simulink model "PolePlacement_Discrete"  (R2021a)
settings: Solver=VariableStepAuto  StartTime=0.0  StopTime=10.0  RelTol=1e-3
values from neighbouring files (symbols this model uses):
  k = place(A, B, new_pole)    [PolePlacement_Controller_script.m]
  k2 = place(sysest.A, sysest.B, new_pole2)    [PolePlacement_Controller_script.m]
  Kr = 1/Kdc(1)    [PolePlacement_Controller_script.m]
  Kr2 = 1/Kdc2    [PolePlacement_Controller_script.m]
  L = place(sysestc.A',sysestc.C', 10*new_pole)'    [PolePlacement_Controller_script.m]
  L22 = place(sysest.A',sysest.C', new_pole2/0.99)'    [PolePlacement_Controller_script.m]
  sysest = load("sysest09c_trick.mat").sysest    [Compensator_schemes.m]    (also in LQGR_Controller_script.m; PolePlacement_Controller_script.m)
undefined symbols (not defined in the file or in its folder): DiscIntNeverNeededParam, sigbuilder_block, sysestc
libraries: cstblocks x2, slpidlib x1
settings Model: Creator=jesuc  LastModifiedBy=andre

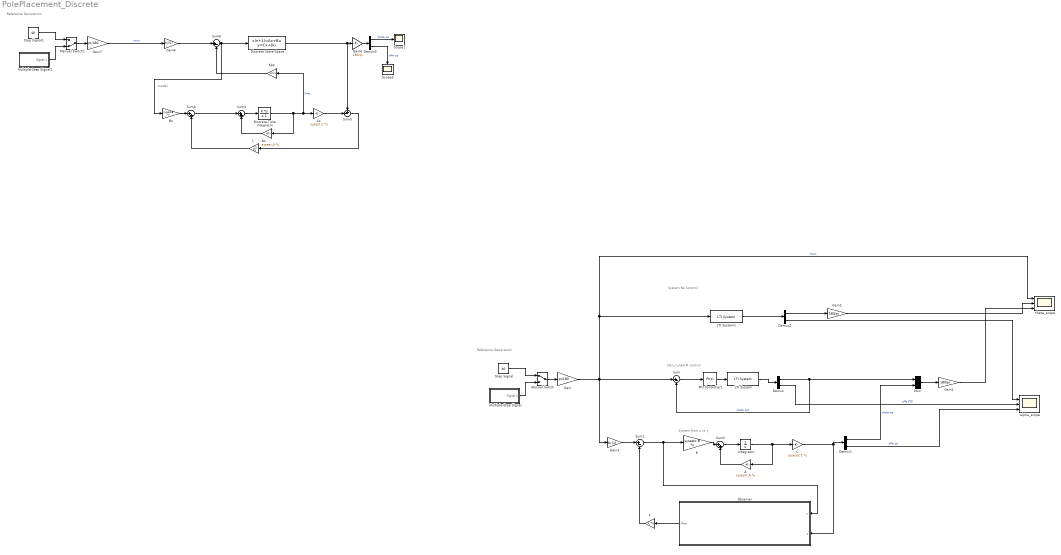
== system PolePlacement_Discrete ==
  note: Non_tuned PI control
  note: System No Control
  note: Reference Generation
  note: System from u to y
  note: model
  note: Reference Generation
  A : Gain  Gain=sysestc.A  Multiplication=Matrix(K*u)
  Ao : Gain  Gain=sysest.A  Multiplication=Matrix(K*u)
  B : Gain  Gain=sysestc.B  Multiplication=Matrix(K*u)
  Bo : Gain  Gain=sysest.B  Multiplication=Matrix(K*u)
  C : Gain  Gain=sysestc.C  Multiplication=Matrix(K*u)
  Co : Gain  Gain=sysest.C  Multiplication=Matrix(K*u)
  Demux{,1..3} (4 alike) : Demux  Outputs=2
  Discrete State-Space : DiscreteStateSpace  A=sysest.A  B=sysest.B  C=sysest.C  D=sysest.D  SampleTime=0.002
  Discrete-Time Integrator : DiscreteIntegrator  SampleTime=0.002  ICPrevOutput=DiscIntNeverNeededParam  ICPrevScaledInput=DiscIntNeverNeededParam
  Gain : Gain  Gain=pi/180
  Gain1 : Gain  Gain=180/pi
  Gain2 : Gain  Gain=180/pi
  Gain3 : Gain  Gain=Kr(1)
  Gain4 : Gain  Gain=Kr2(1)
  Gain6 : Gain  Gain=180/pi
  Gain7 : Gain  Gain=pi/180
  Integrator : Integrator
  K : Gain  Gain=k  Multiplication=Matrix(K*u)
  Kpp : Gain  Gain=k2  Multiplication=Matrix(K*u)
  L : Gain  Gain=L22  Multiplication=Matrix(K*u)
  LTI System : cstblocks/LTI System  sys=tf(sysestc)  IC=[]
  LTI System1 : cstblocks/LTI System  sys=tf(sysestc)  IC=[]
  Manual Switch : ManualSwitch
  Manual Switch1 : ManualSwitch  CurrentSetting=0
  Multiple-Step Signal : Subsystem  Tag=STV Subsys  LoadFcn=sigbuilder_block('load');  StartFcn=sigbuilder_block('start');  StopFcn=sigbuilder_block('stop');  ClipboardFcn=sigbuilder_block('clipboard');  mask(Sigbuilder block){tuvar=[0:10]}
      mask help: Simulink:masks:SigbuilderBlock_MD
      mask init:
      | if ~strcmp(get_param(bdroot(gcbh),'SimulationStatus'),'stopped') tuvar = sigbuilder_block('maskInit'); end
      settings: CopyFcn=sigbuilder_block('copy');  DeleteFcn=sigbuilder_block('delete');  ModelCloseFcn=sigbuilder_block('modelClose');  PreSaveFcn=sigbuilder_block('preSave');  PauseFcn=sigbuilder_block('pause');  ContinueFcn=sigbuilder_block('continue');  NameChangeFcn=sigbuilder_block('namechange');  OpenFcn=sigbuilder_block('open',[437.6 199.2 550.4 400 ]);  CloseFcn=sigbuilder_block('close');
      mask Display: plot(0, 0, 100, 100,[2, 2, 32, 32, 2], [68, 8, 8, 68, 68],[32, 2], [38, 38], [32, 19, 2],[53, 60, 44], [32, 17, 17, 2],[16, 16, 31, 31]);txt = getActiveGroup(gcbh);text(2, 100, txt,'verticalAlignment', 'top');
  Multiple-Step Signal1 : Subsystem  Tag=STV Subsys  LoadFcn=sigbuilder_block('load');  StartFcn=sigbuilder_block('start');  StopFcn=sigbuilder_block('stop');  ClipboardFcn=sigbuilder_block('clipboard');  mask(Sigbuilder block){tuvar=[0:10]}
      mask help: Simulink:masks:SigbuilderBlock_MD
      mask init:
      | if ~strcmp(get_param(bdroot(gcbh),'SimulationStatus'),'stopped') tuvar = sigbuilder_block('maskInit'); end
      settings: CopyFcn=sigbuilder_block('copy');  DeleteFcn=sigbuilder_block('delete');  ModelCloseFcn=sigbuilder_block('modelClose');  PreSaveFcn=sigbuilder_block('preSave');  PauseFcn=sigbuilder_block('pause');  ContinueFcn=sigbuilder_block('continue');  NameChangeFcn=sigbuilder_block('namechange');  OpenFcn=sigbuilder_block('open',[437.6 199.2 550.4 400 ]);  CloseFcn=sigbuilder_block('close');
      mask Display: plot(0, 0, 100, 100,[2, 2, 32, 32, 2], [68, 8, 8, 68, 68],[32, 2], [38, 38], [32, 19, 2],[53, 60, 44], [32, 17, 17, 2],[16, 16, 31, 31]);txt = getActiveGroup(gcbh);text(2, 100, txt,'verticalAlignment', 'top');
  Mux : Mux  Inputs=2
  Observer : Subsystem
  PID Controller1 : slpidlib/PID Controller  Controller=PI  Form=Parallel  TimeDomain=Continuous-time  UseExternalTs=off  SampleTime=-1  IntegratorMethod=Forward Euler  FilterMethod=Forward Euler  ControllerParametersSource=internal  P=1  I=1  D=0  UseFilter=on  N=100  TunerSelectOption=Transfer Function Based (PID Tuner App)  InitialConditionSource=internal  InitialConditionForIntegrator=0  InitialConditionForFilter=0  DifferentiatorICPrevScaledInput=0  ExternalReset=none  TrackingMode=off  Kt=1  LimitOutput=off  SatLimitsSource=internal  UpperSaturationLimit=inf  LowerSaturationLimit=-inf  LinearizeAsGain=on  AntiWindupMode=none  Kb=1  POutMin=[]  POutMax=[]  IOutMin=[]  IOutMax=[]  DOutMin=[]  DOutMax=[]  NOutMin=[]  NOutMax=[]  SumOutMin=[]  SumOutMax=[]  SaturationOutMin=[]  SaturationOutMax=[]  PParamMin=[]  PParamMax=[]  IParamMin=[]  IParamMax=[]  DParamMin=[]  DParamMax=[]  NParamMin=[]  NParamMax=[]  KbParamMin=[]  KbParamMax=[]  KtParamMin=[]  KtParamMax=[]  KbOutMin=[]  KbOutMax=[]  KtOutMin=[]  KtOutMax=[]  IntegratorOutMin=[]  IntegratorOutMax=[]  FilterOutMin=[]  FilterOutMax=[]  SumI1OutMin=[]  SumI1OutMax=[]  SumI2OutMin=[]  SumI2OutMax=[]  SumI3OutMin=[]  SumI3OutMax=[]  SumI4OutMin=[]  SumI4OutMax=[]  SumDOutMin=[]  SumDOutMax=[]  DifferentiatorOutMin=[]  DifferentiatorOutMax=[]  FilterDiffOutCoefMin=[]  FilterDiffOutCoefMax=[]  ReciprocalOutMin=[]  ReciprocalOutMax=[]  SumDenOutMin=[]  SumDenOutMax=[]  SumNumOutMin=[]  SumNumOutMax=[]  DivideOutMin=[]  DivideOutMax=[]  UdiffTsProdOutMin=[]  UdiffTsProdOutMax=[]  NTsProdOutMin=[]  NTsProdOutMax=[]  UintegralTsProdOutMin=[]  UintegralTsProdOutMax=[]  UngainTsProdOutMin=[]  UngainTsProdOutMax=[]  IntegratorContinuousStateAttributes=''  IntegratorStateMustResolveToSignalObject=off  IntegratorRTWStateStorageClass=Auto  FilterContinuousStateAttributes=''  FilterStateMustResolveToSignalObject=off  FilterRTWStateStorageClass=Auto  ParallelPVariant=InternalParameters  IdealPVariant=Disabled  IVariant=InternalParameters  DVariant=Disabled  IntegratorVariant=Continuous  SatVariant=Disabled  AWVariant=Passthrough  PCopyVariant=Disabled  TRVariant=Disabled  FdbkBlocksVariant=Forward  IdealPFdbkVariant=Disabled  SatFdbkVariant=Disabled  DerivativeFilterVariant=Disabled  NVariant=Disabled  NCopyVariant=Disabled_SignalSpec  FilterICVariant=Disabled  IntegratorICVariant=InternalICs  ExternalResetVariant=Disabled  TRSumVariant=Passthrough  SumFdbkVariant=Disabled  SumVariant=Sum_PI  TsampFilterVariant=InternalTs  TsampNgainVariant=Passthrough  TsampIntegralVariant=Passthrough  ExternalSaturationOutDataTypeStr=Inherit: Same as second input
  Scope1 : Scope
  Scope3 : Scope
  Step Signal : Constant  Value=40
  Step Signal1 : Constant  Value=40
  Sum : Sum  Inputs=|+-
  Sum1 : Sum  Inputs=|+-
  Sum2 : Sum  Inputs=|++
  Sum3 : Sum  Inputs=|++
  Sum4 : Sum  Inputs=|++
  Sum5 : Sum  Inputs=+-|
  Sum6 : Sum  Inputs=|+-
  alpha_scope : Scope  NumInputPorts=3
  theta_scope : Scope  NumInputPorts=3
  wires:
  Gain/1 -> theta_scope/1, LTI System1/1, Sum/1, Gain3/1  "input"
  Sum/1 -> PID Controller1/1
  PID Controller1/1 -> LTI System/1
  LTI System/1 -> Demux/1
  Demux/1 -> Sum/2, Mux/1  "theta pid"
  B/1 -> Sum2/1
  Sum2/1 -> Integrator/1
  Integrator/1 -> A/1, C/1
  A/1 -> Sum2/2
  K/1 -> Sum1/2
  C/1 -> Demux1/1, Observer/2(y)
  Demux1/1 -> Mux/2  "theta pp"
  Demux1/2 -> alpha_scope/3  "alfa pp"
  Gain3/1 -> Sum1/1
  Demux/2 -> alpha_scope/2  "alfa PID"
  Gain1/1 -> theta_scope/3
  Mux/1 -> Gain1/1
  Sum1/1 -> Observer/1(u), B/1
  Observer/1(Xhat) -> K/1
  LTI System1/1 -> Demux2/1
  Demux2/1 -> Gain2/1
  Gain2/1 -> theta_scope/2
  Demux2/2 -> alpha_scope/1
  Demux3/1 -> Scope1/1  "theta pp"
  Kpp/1 -> Sum6/2
  Sum4/1 -> Sum3/1
  Sum3/1 -> Discrete-Time Integrator/1
  Bo/1 -> Sum4/1
  Co/1 -> Sum5/2
  Gain4/1 -> Sum6/1
  Ao/1 -> Sum3/2
  L/1 -> Sum4/2
  Discrete-Time Integrator/1 -> Ao/1, Kpp/1, Co/1  "Xhat"
  Discrete State-Space/1 -> Gain6/1, Sum5/1
  Sum5/1 -> L/1
  Sum6/1 -> Discrete State-Space/1, Bo/1
  Demux3/2 -> Scope3/1  "alfa pp"
  Gain6/1 -> Demux3/1
  Multiple-Step Signal/1(Signal 1) -> Manual Switch/2
  Manual Switch/1 -> Gain/1
  Step Signal/1 -> Manual Switch/1
  Manual Switch1/1 -> Gain7/1
  Step Signal1/1 -> Manual Switch1/1
  Multiple-Step Signal1/1(Signal 1) -> Manual Switch1/2
  Gain7/1 -> Gain4/1  "input"

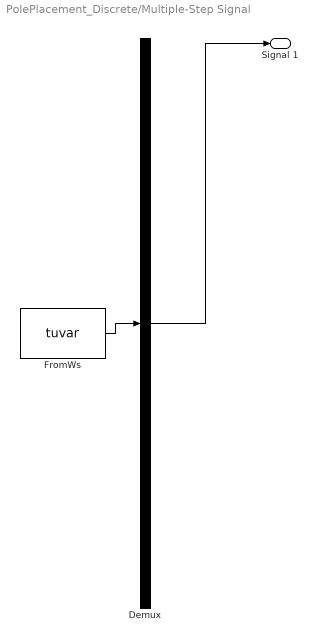
== system PolePlacement_Discrete/Multiple-Step Signal ==
  Demux : Demux  Tag=STV Demux  Outputs=1
      settings: DisplayOption=none
  FromWs : FromWorkspace  Tag=STV FromWs  VariableName=tuvar
      SigBuilderData=|
      | common.afterFinalStr = 'Extrapolate'
      | common.sampleTime = 0
      | dataSet.timeRange = [0 10]
      | dataSet.name = 'Group 1'
      | sbobj.Groups.Name = 'Group 1'
      | sbobj.Groups.Signals.Name = 'Signal 1'
      | sbobj.Groups.Signals.XData = [0 1 1 3 3 5 5 7 7 8.5 8.5 10]
      | sbobj.Groups.Signals.YData = [0.005 0.005 40 40 15 15 -30 -30 0 0 23 23]
  Signal 1 : Outport  Tag=STV Outport
  wires:
  Demux/1 -> Signal 1/1
  FromWs/1 -> Demux/1

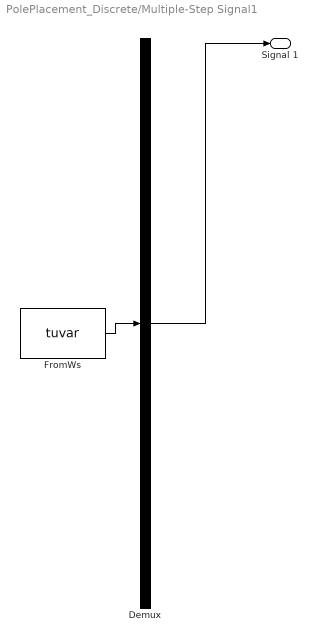
== system PolePlacement_Discrete/Multiple-Step Signal1 ==
  Demux : Demux  Tag=STV Demux  Outputs=1
      settings: DisplayOption=none
  FromWs : FromWorkspace  Tag=STV FromWs  VariableName=tuvar
      SigBuilderData=|
      | common.afterFinalStr = 'Extrapolate'
      | common.sampleTime = 0
      | dataSet.timeRange = [0 10]
      | dataSet.name = 'Group 1'
      | sbobj.Groups.Name = 'Group 1'
      | sbobj.Groups.Signals.Name = 'Signal 1'
      | sbobj.Groups.Signals.XData = [0 1 1 3 3 5 5 7 7 8.5 8.5 10]
      | sbobj.Groups.Signals.YData = [0.005 0.005 40 40 15 15 -30 -30 0 0 23 23]
  Signal 1 : Outport  Tag=STV Outport
  wires:
  Demux/1 -> Signal 1/1
  FromWs/1 -> Demux/1

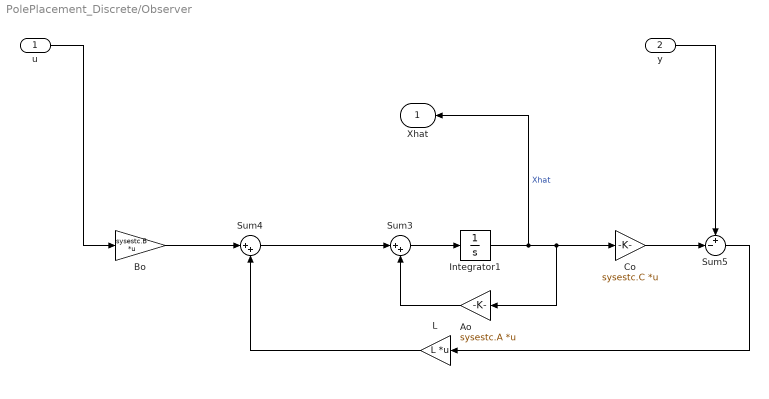
== system PolePlacement_Discrete/Observer ==
  u : Inport
  y : Inport  Port=2
  Ao : Gain  Gain=sysestc.A  Multiplication=Matrix(K*u)
  Bo : Gain  Gain=sysestc.B  Multiplication=Matrix(K*u)
  Co : Gain  Gain=sysestc.C  Multiplication=Matrix(K*u)
  Integrator1 : Integrator
  L : Gain  Gain=L  Multiplication=Matrix(K*u)
  Sum3 : Sum  Inputs=|++
  Sum4 : Sum  Inputs=|++
  Sum5 : Sum  Inputs=+-|
  Xhat : Outport
  wires:
  Sum5/1 -> L/1
  Sum4/1 -> Sum3/1
  u/1 -> Bo/1
  Sum3/1 -> Integrator1/1
  Integrator1/1 -> Xhat/1, Ao/1, Co/1  "Xhat"
  Ao/1 -> Sum3/2
  L/1 -> Sum4/2
  Co/1 -> Sum5/2
  Bo/1 -> Sum4/1
  y/1 -> Sum5/1
